simulink model "svpwm"  (R2015a)
settings: Solver=ode3  StartTime=0.0  StopTime=0.06  FixedStep=2e-6  MaxStep=0.00001  RelTol=1e-3
libraries: powerlib x13, dspsrcs4 x3, simulink x2
settings Model: Creator=Administrator  LastModifiedBy=think0404
settings DebuggingCC: UnderspecifiedInitializationDetection=Classic  MergeDetectMultiDrivingBlocksExec=none  SolverPrmCheckMsg=warning  StateNameClashWarn=warning

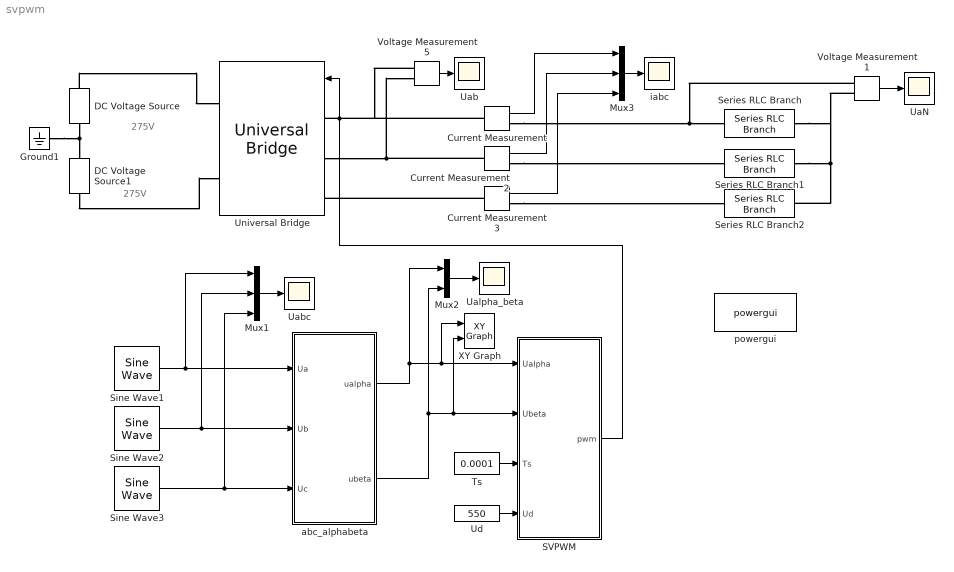
== system svpwm ==
  note: 275V
  note: 275V
  Current Measurement : powerlib/Measurements/Current Measurement  PhasorSimulation=off  OutputType=Complex  PSBequivalent=0
  Current Measurement2 : powerlib/Measurements/Current Measurement  PhasorSimulation=off  OutputType=Complex  PSBequivalent=0
  Current Measurement3 : powerlib/Measurements/Current Measurement  PhasorSimulation=off  OutputType=Complex  PSBequivalent=0
  DC Voltage Source : powerlib/Electrical Sources/DC Voltage Source  Amplitude=275  Measurements=None
  DC Voltage Source1 : powerlib/Electrical Sources/DC Voltage Source  Amplitude=275  Measurements=None
  Ground1 : powerlib/Elements/Ground  LConnTagsString=a
  Mux1 : Mux  Inputs=3
  Mux2 : Mux  Inputs=2
  Mux3 : Mux  Inputs=3
  SVPWM : Subsystem
  Series RLC Branch : powerlib/Elements/Series RLC Branch  LConnTagsString=__new0  RConnTagsString=__new0  BranchType=RL  Resistance=1  Inductance=1e-3  SetiL0=off  InitialCurrent=0  Capacitance=1e-6  Setx0=off  InitialVoltage=0  Measurements=None
  Series RLC Branch1 : powerlib/Elements/Series RLC Branch  LConnTagsString=__new0  RConnTagsString=__new0  BranchType=RL  Resistance=1  Inductance=1e-3  SetiL0=off  InitialCurrent=0  Capacitance=1e-6  Setx0=off  InitialVoltage=0  Measurements=None
  Series RLC Branch2 : powerlib/Elements/Series RLC Branch  LConnTagsString=__new0  RConnTagsString=__new0  BranchType=RL  Resistance=1  Inductance=1e-3  SetiL0=off  InitialCurrent=0  Capacitance=1e-6  Setx0=off  InitialVoltage=0  Measurements=None
  Sine Wave1 : dspsrcs4/Sine Wave  Amplitude=311  Frequency=50  Phase=0  SampleMode=Discrete  OutComplex=Real  CompMethod=Trigonometric fcn  TableSize=Speed  SampleTime=2e-6  SamplesPerFrame=1  ResetState=Restart at time zero  dataType=double  wordLen=16  udDataType=sfix(16)  fracBitsMode=Best precision  numFracBits=15  OutDataTypeStr=double  LastOutDataTypeStr=double
  Sine Wave2 : dspsrcs4/Sine Wave  Amplitude=311  Frequency=50  Phase=-2*pi/3  SampleMode=Discrete  OutComplex=Real  CompMethod=Trigonometric fcn  TableSize=Speed  SampleTime=2e-6  SamplesPerFrame=1  ResetState=Restart at time zero  dataType=double  wordLen=16  udDataType=sfix(16)  fracBitsMode=Best precision  numFracBits=15  OutDataTypeStr=double  LastOutDataTypeStr=double
  Sine Wave3 : dspsrcs4/Sine Wave  Amplitude=311  Frequency=50  Phase=-4*pi/3  SampleMode=Discrete  OutComplex=Real  CompMethod=Trigonometric fcn  TableSize=Speed  SampleTime=2e-6  SamplesPerFrame=1  ResetState=Restart at time zero  dataType=double  wordLen=16  udDataType=sfix(16)  fracBitsMode=Best precision  numFracBits=15  OutDataTypeStr=double  LastOutDataTypeStr=double
  Ts : Constant  Value=0.0001
  UaN : Scope
      settings: SaveName=ScopeData6
  Uab : Scope
      settings: YMin=-600  YMax=600
  Uabc : Scope
      settings: YMin=-35  YMax=35  SaveName=ScopeData7
  Ualpha_beta : Scope
      settings: YMin=-1.1e+006  YMax=1.1e+006  SaveName=ScopeData4
  Ud : Constant  Value=550
  Universal Bridge : powerlib/Power Electronics/Universal Bridge  Arms=3  SnubberResistance=1e5  SnubberCapacitance=inf  Device=MOSFET / Diodes  Ron=1e-3  Lon=0  ForwardVoltages="[  0  0  ]"  ForwardVoltage=0  GTOparameters=[ 10e-6 , 20e-6 ]  IGBTparameters=[ 1e-6 , 2e-6 ]  Measurements=None  Measurements_2=None  converterType=Rectifier
  Voltage Measurement1 : powerlib/Measurements/Voltage Measurement  PhasorSimulation=off  OutputType=Complex  PSBequivalent=0
  Voltage Measurement5 : powerlib/Measurements/Voltage Measurement  PhasorSimulation=off  OutputType=Complex  PSBequivalent=0
  XY Graph : simulink/Sinks/XY Graph  xmin=-550  xmax=550  ymin=-550  ymax=550  st=-1
  abc_alphabeta : Subsystem
  iabc : Scope
      settings: YMin=-300  YMax=300  SaveName=ScopeData5
  powergui : powerlib/powergui  Priority=1  SimulationMode=Discrete  SolverType=Tustin  SampleTime=2e-6  frequency=60  SPID=off  DisableSnubberDevices=off  DisableRonSwitches=off  DisableVfSwitches=off  SwTol=0  DisplayEquations=off  Interpol=off  methode=off  Ts=0  FunctionMessages=off  echomessages=off  HookPort=off  EnableUseOfTLC=off  x0status=blocks  frequencyindice=0  Pbase=100e6  ErrMax=1e-4  Iterations=50  UnitsV=kV  UnitsW=MW  buscounter=0  RestoreLinks=warning  ResistiveCurrentMeasurement=off  Frange=[0:2:500]  Ylog=off  Xlog=on  ShowGrid=off  save=off  variable=ZData  structure=0  ZoomFFT=off  StartTime=0.0  cycles=1  DisplayStyle=1  fundamental=60  FreqAxis=off  MaxFrequency=1000  frequencyindicesteady=1  RmsSteady=1  display=off
  wires:
  Ts/1 -> SVPWM/3(Ts)
  Ud/1 -> SVPWM/4(Ud)
  Mux2/1 -> Ualpha_beta/1
  SVPWM/1(pwm) -> Universal Bridge/1
  Voltage Measurement5/1 -> Uab/1
  Voltage Measurement1/1 -> UaN/1
  Mux1/1 -> Uabc/1
  Sine Wave1/1 -> Mux1/1, abc_alphabeta/1(Ua)
  Sine Wave2/1 -> Mux1/2, abc_alphabeta/2(Ub)
  Sine Wave3/1 -> Mux1/3, abc_alphabeta/3(Uc)
  abc_alphabeta/1(ualpha) -> Mux2/1, XY Graph/1, SVPWM/1(Ualpha)
  abc_alphabeta/2(ubeta) -> Mux2/2, XY Graph/2, SVPWM/2(Ubeta)
  Mux3/1 -> iabc/1
  Current Measurement/1 -> Mux3/1
  Current Measurement2/1 -> Mux3/2
  Current Measurement3/1 -> Mux3/3
  connections:
  Current Measurement3/LConn1 -- Universal Bridge/LConn3
  DC Voltage Source/RConn1 -- Universal Bridge/RConn1
  DC Voltage Source/LConn1 -- DC Voltage Source1/RConn1 -- Ground1/LConn1
  DC Voltage Source1/LConn1 -- Universal Bridge/RConn2
  Universal Bridge/LConn1 -- Current Measurement/LConn1 -- Voltage Measurement5/LConn1
  Universal Bridge/LConn2 -- Current Measurement2/LConn1 -- Voltage Measurement5/LConn2
  Series RLC Branch1/RConn1 -- Series RLC Branch2/RConn1 -- Voltage Measurement1/LConn2 -- Series RLC Branch/RConn1
  Current Measurement/RConn1 -- Series RLC Branch/LConn1 -- Voltage Measurement1/LConn1
  Current Measurement2/RConn1 -- Series RLC Branch1/LConn1
  Current Measurement3/RConn1 -- Series RLC Branch2/LConn1

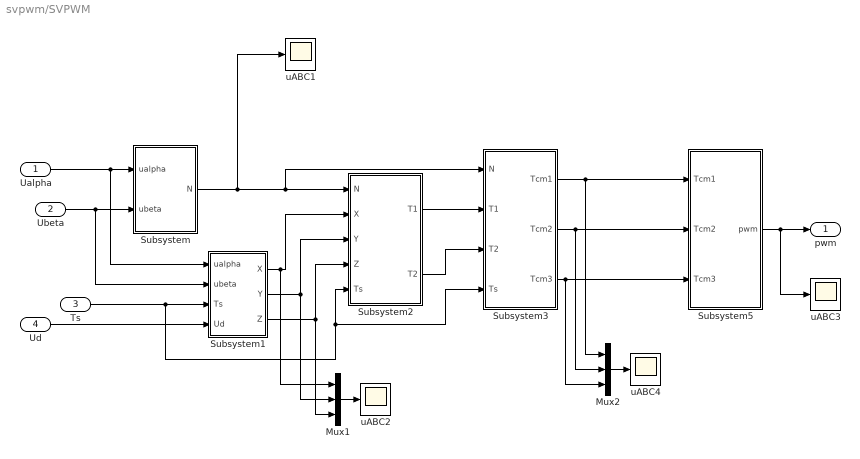
== system svpwm/SVPWM ==
  Ualpha : Inport
  Ubeta : Inport  Port=2
  Ts : Inport  Port=3
  Ud : Inport  Port=4
  Mux1 : Mux  Inputs=3
  Mux2 : Mux  Inputs=3
  Subsystem : Subsystem
  Subsystem1 : Subsystem
  Subsystem2 : Subsystem
  Subsystem3 : Subsystem
  Subsystem5 : Subsystem
  uABC{1..4} (4 alike) : Scope
      uABC1 settings: YMin=-750  YMax=750  SaveName=ScopeData2
      uABC2 settings: YMin=-750  YMax=750  SaveName=ScopeData3
      uABC3 settings: YMin=0  YMax=1  SaveName=ScopeData10
      uABC4 settings: YMin=-2.5e-006  YMax=5.25e-005
  pwm : Outport
  wires:
  Subsystem/1(N) -> Subsystem2/1(N), Subsystem3/1(N), uABC1/1
  Subsystem1/1(X) -> Subsystem2/2(X), Mux1/1
  Subsystem1/2(Y) -> Subsystem2/3(Y), Mux1/2
  Subsystem1/3(Z) -> Subsystem2/4(Z), Mux1/3
  Ts/1 -> Subsystem2/5(Ts), Subsystem3/4(Ts), Subsystem1/3(Ts)
  Ualpha/1 -> Subsystem/1(ualpha), Subsystem1/1(ualpha)
  Ubeta/1 -> Subsystem/2(ubeta), Subsystem1/2(ubeta)
  Ud/1 -> Subsystem1/4(Ud)
  Subsystem2/1(T1) -> Subsystem3/2(T1)
  Subsystem2/2(T2) -> Subsystem3/3(T2)
  Subsystem3/1(Tcm1) -> Mux2/1, Subsystem5/1(Tcm1)
  Subsystem3/2(Tcm2) -> Mux2/2, Subsystem5/2(Tcm2)
  Subsystem3/3(Tcm3) -> Mux2/3, Subsystem5/3(Tcm3)
  Mux1/1 -> uABC2/1
  Subsystem5/1(pwm) -> pwm/1, uABC3/1
  Mux2/1 -> uABC4/1

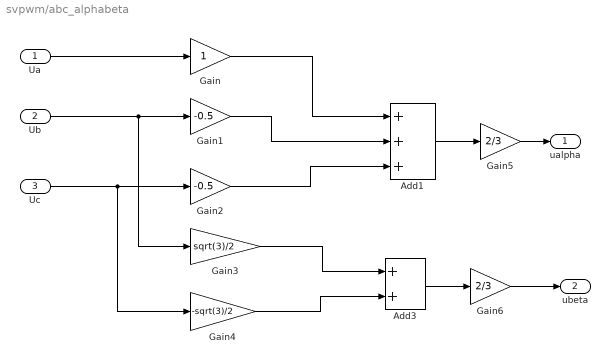
== system svpwm/abc_alphabeta ==
  Ua : Inport
  Ub : Inport  Port=2
  Uc : Inport  Port=3
  Add1 : Sum  Inputs=+++
  Add3 : Sum
  Gain : Gain
  Gain1 : Gain  Gain=-0.5
  Gain2 : Gain  Gain=-0.5
  Gain3 : Gain  Gain=sqrt(3)/2
  Gain4 : Gain  Gain=-sqrt(3)/2
  Gain5 : Gain  Gain=2/3
  Gain6 : Gain  Gain=2/3
  ualpha : Outport
  ubeta : Outport  Port=2
  wires:
  Add1/1 -> Gain5/1
  Add3/1 -> Gain6/1
  Ua/1 -> Gain/1
  Ub/1 -> Gain3/1, Gain1/1
  Uc/1 -> Gain4/1, Gain2/1
  Gain/1 -> Add1/1
  Gain1/1 -> Add1/2
  Gain2/1 -> Add1/3
  Gain3/1 -> Add3/1
  Gain4/1 -> Add3/2
  Gain5/1 -> ualpha/1
  Gain6/1 -> ubeta/1

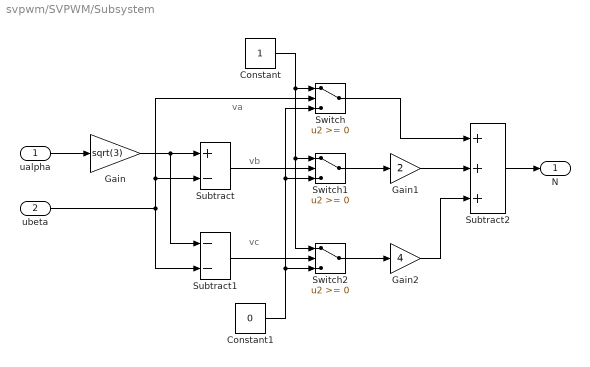
== system svpwm/SVPWM/Subsystem ==
  note: vb
  note: va
  note: vc
  ualpha : Inport
  ubeta : Inport  Port=2
  Constant : Constant
  Constant1 : Constant  Value=0
  Gain : Gain  Gain=sqrt(3)
  Gain1 : Gain  Gain=2
  Gain2 : Gain  Gain=4
  Subtract : Sum  Inputs=+-
  Subtract1 : Sum  Inputs=--
  Subtract2 : Sum  Inputs=+++
  Switch : Switch
  Switch1 : Switch
  Switch2 : Switch
  N : Outport
  wires:
  Gain/1 -> Subtract/1, Subtract1/1
  ualpha/1 -> Gain/1
  ubeta/1 -> Subtract/2, Switch/2, Subtract1/2
  Subtract/1 -> Switch1/2
  Subtract1/1 -> Switch2/2
  Constant/1 -> Switch/1, Switch1/1, Switch2/1
  Constant1/1 -> Switch2/3, Switch1/3, Switch/3
  Switch1/1 -> Gain1/1
  Switch2/1 -> Gain2/1
  Gain1/1 -> Subtract2/2
  Switch/1 -> Subtract2/1
  Gain2/1 -> Subtract2/3
  Subtract2/1 -> N/1

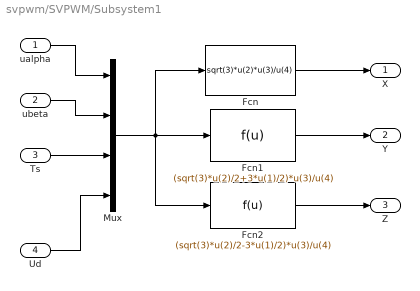
== system svpwm/SVPWM/Subsystem1 ==
  ualpha : Inport
  ubeta : Inport  Port=2
  Ts : Inport  Port=3
  Ud : Inport  Port=4
  Fcn : Fcn  Expr=sqrt(3)*u(2)*u(3)/u(4)
  Fcn1 : Fcn  Expr=(sqrt(3)*u(2)/2+3*u(1)/2)*u(3)/u(4)
  Fcn2 : Fcn  Expr=(sqrt(3)*u(2)/2-3*u(1)/2)*u(3)/u(4)
  Mux : Mux
  X : Outport
  Y : Outport  Port=2
  Z : Outport  Port=3
  wires:
  Ud/1 -> Mux/4
  ualpha/1 -> Mux/1
  ubeta/1 -> Mux/2
  Ts/1 -> Mux/3
  Fcn/1 -> X/1
  Fcn1/1 -> Y/1
  Fcn2/1 -> Z/1
  Mux/1 -> Fcn/1, Fcn1/1, Fcn2/1

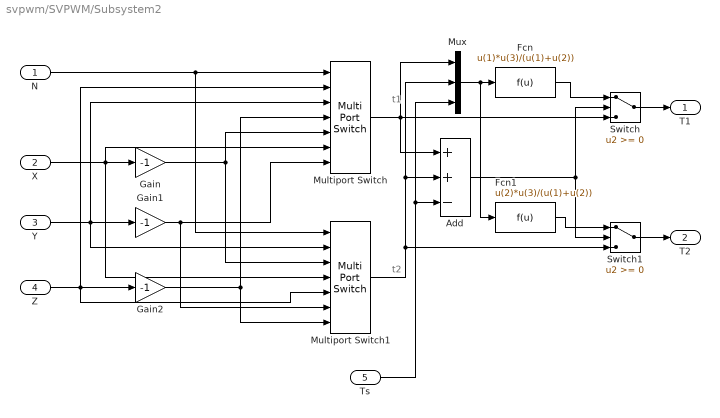
== system svpwm/SVPWM/Subsystem2 ==
  note: t1
  note: t2
  N : Inport
  X : Inport  Port=2
  Y : Inport  Port=3
  Z : Inport  Port=4
  Ts : Inport  Port=5
  Add : Sum  Inputs=++-
  Fcn : Fcn  Expr=u(1)*u(3)/(u(1)+u(2))
  Fcn1 : Fcn  Expr=u(2)*u(3)/(u(1)+u(2))
  Gain : Gain  Gain=-1
  Gain1 : Gain  Gain=-1
  Gain2 : Gain  Gain=-1
  Multiport Switch : MultiPortSwitch  Inputs=6
  Multiport Switch1 : MultiPortSwitch  Inputs=6
  Mux : Mux  Inputs=3
  Switch : Switch
  Switch1 : Switch
  T1 : Outport
  T2 : Outport  Port=2
  wires:
  Z/1 -> Gain2/1, Multiport Switch/2, Multiport Switch1/5
  Y/1 -> Gain1/1, Multiport Switch1/2, Multiport Switch/3
  X/1 -> Multiport Switch1/4, Multiport Switch/6, Gain/1
  N/1 -> Multiport Switch/1, Multiport Switch1/1
  Gain/1 -> Multiport Switch1/3, Multiport Switch/5
  Gain2/1 -> Multiport Switch/4, Multiport Switch1/7
  Gain1/1 -> Multiport Switch1/6, Multiport Switch/7
  Multiport Switch/1 -> Add/1, Mux/1, Switch/3
  Multiport Switch1/1 -> Add/2, Mux/2, Switch1/3
  Ts/1 -> Add/3, Mux/3
  Add/1 -> Switch1/2, Switch/2
  Mux/1 -> Fcn/1, Fcn1/1
  Fcn/1 -> Switch/1
  Fcn1/1 -> Switch1/1
  Switch/1 -> T1/1
  Switch1/1 -> T2/1

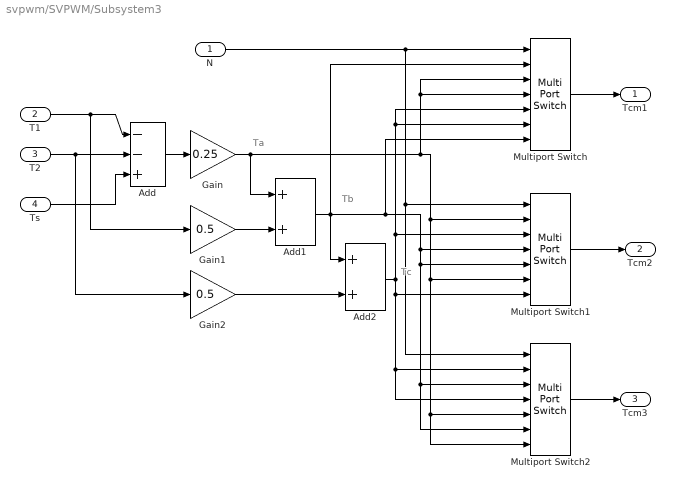
== system svpwm/SVPWM/Subsystem3 ==
  note: Ta
  note: Tb
  note: Tc
  N : Inport
  T1 : Inport  Port=2
  T2 : Inport  Port=3
  Ts : Inport  Port=4
  Add : Sum  Inputs=--+
  Add1 : Sum
  Add2 : Sum
  Gain : Gain  Gain=0.25
  Gain1 : Gain  Gain=0.5
  Gain2 : Gain  Gain=0.5
  Multiport Switch : MultiPortSwitch  Inputs=6
  Multiport Switch1 : MultiPortSwitch  Inputs=6
  Multiport Switch2 : MultiPortSwitch  Inputs=6
  Tcm1 : Outport
  Tcm2 : Outport  Port=2
  Tcm3 : Outport  Port=3
  wires:
  T1/1 -> Add/1, Gain1/1
  T2/1 -> Add/2, Gain2/1
  Ts/1 -> Add/3
  Add/1 -> Gain/1
  Gain/1 -> Add1/1, Multiport Switch/3, Multiport Switch/4, Multiport Switch1/2, Multiport Switch1/6, Multiport Switch2/5, Multiport Switch2/7
  Gain1/1 -> Add1/2
  Add1/1 -> Multiport Switch/2, Add2/1, Multiport Switch1/4, Multiport Switch1/5, Multiport Switch2/6, Multiport Switch2/3, Multiport Switch/7
  Gain2/1 -> Add2/2
  N/1 -> Multiport Switch/1, Multiport Switch1/1, Multiport Switch2/1
  Add2/1 -> Multiport Switch1/3, Multiport Switch/5, Multiport Switch/6, Multiport Switch2/2, Multiport Switch2/4, Multiport Switch1/7
  Multiport Switch/1 -> Tcm1/1
  Multiport Switch1/1 -> Tcm2/1
  Multiport Switch2/1 -> Tcm3/1

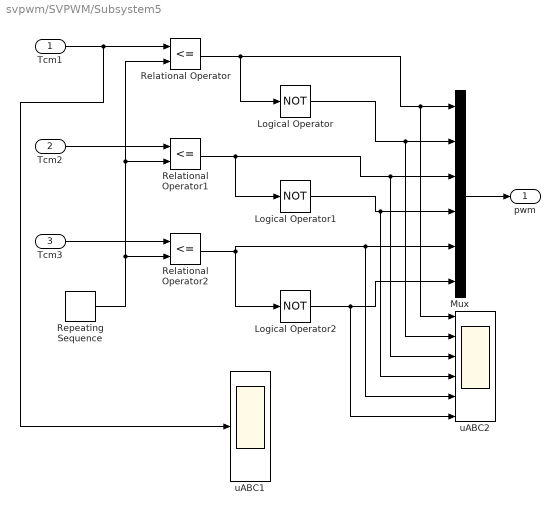
== system svpwm/SVPWM/Subsystem5 ==
  Tcm1 : Inport
  Tcm2 : Inport  Port=2
  Tcm3 : Inport  Port=3
  Logical Operator : Logic  Operator=NOT  AllPortsSameDT=off  OutDataTypeStr=boolean
  Logical Operator1 : Logic  Operator=NOT  AllPortsSameDT=off  OutDataTypeStr=boolean
  Logical Operator2 : Logic  Operator=NOT  AllPortsSameDT=off  OutDataTypeStr=boolean
  Mux : Mux  Inputs=6
  Relational Operator : RelationalOperator  Operator=<=  OutDataTypeStr=boolean
  Relational Operator1 : RelationalOperator  Operator=<=  OutDataTypeStr=boolean
  Relational Operator2 : RelationalOperator  Operator=<=  OutDataTypeStr=boolean
  Repeating Sequence : simulink/Sources/Repeating Sequence  rep_seq_t=[0 5e-5 1e-4]  rep_seq_y=[0 5e-5 0]
  uABC1 : Scope
      settings: YMin=1e-05  YMax=4e-05  SaveName=ScopeData33
  uABC2 : Scope  NumInputPorts=6
      settings: YMin=-750~-5~-5~-5~-5~-5  YMax=750~5~5~5~5~5  SaveName=ScopeData9
  pwm : Outport
  wires:
  Tcm1/1 -> uABC1/1, Relational Operator/1
  Tcm2/1 -> Relational Operator1/1
  Tcm3/1 -> Relational Operator2/1
  Repeating Sequence/1 -> Relational Operator2/2, Relational Operator1/2, Relational Operator/2
  Relational Operator/1 -> Logical Operator/1, Mux/1, uABC2/1
  Relational Operator1/1 -> Logical Operator1/1, Mux/3, uABC2/3
  Relational Operator2/1 -> Logical Operator2/1, Mux/5, uABC2/5
  Mux/1 -> pwm/1
  Logical Operator/1 -> Mux/2, uABC2/2
  Logical Operator1/1 -> Mux/4, uABC2/4
  Logical Operator2/1 -> Mux/6, uABC2/6
